simulink library "quat2RotMat_ul"  (R2018b)
settings: Solver=VariableStepAuto  StartTime=0.0  StopTime=10.0  RelTol=1e-3
libraries: sharedutil x1
settings Model: Creator=mcobb  LastModifiedBy=mcobb

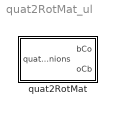
== system quat2RotMat_ul ==
  quat2RotMat : Subsystem

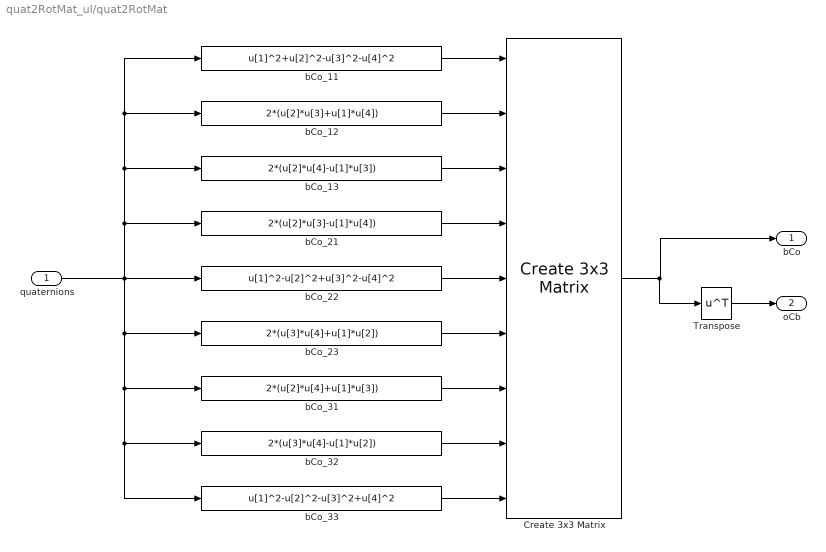
== system quat2RotMat_ul/quat2RotMat ==
  quaternions : Inport
  Create 3x3 Matrix : sharedutil/Create 3x3 Matrix  aMode=aMode
  Transpose : Math  Operator=transpose  SaturateOnIntegerOverflow=on
  bCo_11 : Fcn  Expr=u[1]^2+u[2]^2-u[3]^2-u[4]^2
  bCo_12 : Fcn  Expr=2*(u[2]*u[3]+u[1]*u[4])
  bCo_13 : Fcn  Expr=2*(u[2]*u[4]-u[1]*u[3])
  bCo_21 : Fcn  Expr=2*(u[2]*u[3]-u[1]*u[4])
  bCo_22 : Fcn  Expr=u[1]^2-u[2]^2+u[3]^2-u[4]^2
  bCo_23 : Fcn  Expr=2*(u[3]*u[4]+u[1]*u[2])
  bCo_31 : Fcn  Expr=2*(u[2]*u[4]+u[1]*u[3])
  bCo_32 : Fcn  Expr=2*(u[3]*u[4]-u[1]*u[2])
  bCo_33 : Fcn  Expr=u[1]^2-u[2]^2-u[3]^2+u[4]^2
  bCo : Outport  PortDimensions=[3,3]
  oCb : Outport  Port=2  PortDimensions=[3,3]
  wires:
  Transpose/1 -> oCb/1
  Create 3x3 Matrix/1 -> bCo/1, Transpose/1
  bCo_33/1 -> Create 3x3 Matrix/9
  bCo_32/1 -> Create 3x3 Matrix/8
  bCo_31/1 -> Create 3x3 Matrix/7
  bCo_23/1 -> Create 3x3 Matrix/6
  bCo_22/1 -> Create 3x3 Matrix/5
  bCo_21/1 -> Create 3x3 Matrix/4
  bCo_13/1 -> Create 3x3 Matrix/3
  bCo_12/1 -> Create 3x3 Matrix/2
  bCo_11/1 -> Create 3x3 Matrix/1
  quaternions/1 -> bCo_22/1, bCo_21/1, bCo_13/1, bCo_12/1, bCo_11/1, bCo_23/1, bCo_31/1, bCo_33/1, bCo_32/1
